simulink model "QuarterModelMatrix"  (R2017a)
settings: Solver=FixedStepAuto  StartTime=0.0  StopTime=1.5  FixedStep=1e-3  RelTol=1e-5
values from neighbouring files (symbols this model uses):
  IC = [-1.74412834455962e-12, ... (first row only)    [matrix_main.m]
  step_size = steps_all(i)    [main.m]
undefined symbols (not defined in the file or in its folder): SimFunc
settings Model: Creator=alexkost  LastModifiedBy=alexkost

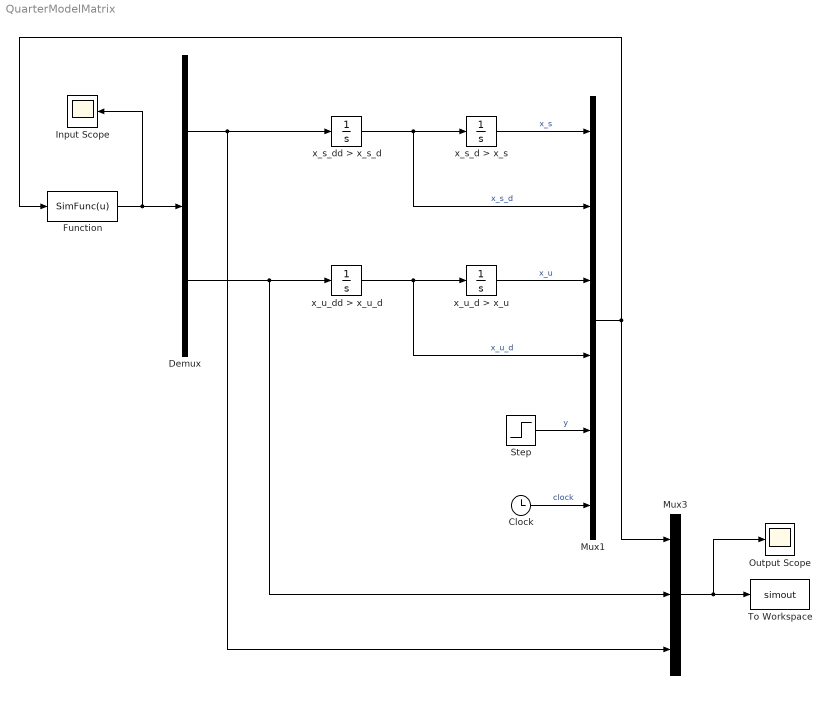
== system QuarterModelMatrix ==
  Clock : Clock
  Demux : Demux  Outputs=2
  Function : MATLABFcn  MATLABFcn=SimFunc(u)
  Input Scope : Scope
  Mux1 : Mux  Inputs=6
  Mux3 : Mux  Inputs=3
  Output Scope : Scope
  Step : Step  Time=0.5  After=step_size  SampleTime=0
  To Workspace : ToWorkspace  VariableName=simout  SampleTime=-1
  x_s_d > x_s : Integrator  InitialCondition=IC(1)
  x_s_dd > x_s_d : Integrator  InitialCondition=IC(2)
  x_u_d > x_u : Integrator  InitialCondition=IC(3)
  x_u_dd > x_u_d : Integrator  InitialCondition=IC(4)
  wires:
  Mux1/1 -> Mux3/1, Function/1
  x_s_dd > x_s_d/1 -> x_s_d > x_s/1, Mux1/2  "x_s_d"
  x_u_d > x_u/1 -> Mux1/3  "x_u"
  x_u_dd > x_u_d/1 -> x_u_d > x_u/1, Mux1/4  "x_u_d"
  Function/1 -> Input Scope/1, Demux/1
  x_s_d > x_s/1 -> Mux1/1  "x_s"
  Demux/2 -> Mux3/2, x_u_dd > x_u_d/1
  Step/1 -> Mux1/5  "y"
  Clock/1 -> Mux1/6  "clock"
  Demux/1 -> Mux3/3, x_s_dd > x_s_d/1
  Mux3/1 -> Output Scope/1, To Workspace/1
